simulink model "test_gps_01"  (Simulink 8.8)
settings: Solver=FixedStepDiscrete  StartTime=0.0  StopTime=10.0  FixedStep=0.001  RelTol=1e-3  EnableMultiTasking=on
InitFcn:
  | px4_ap1_mdl_callback('check_model');
libraries: px4_ap1_px4setup_lib x1, px4_ap1_gps_lib x1
settings Model: Creator=Privat  LastModifiedBy=Privat
settings OptimizationCC: ExpressionDepthLimit=2147483647  InitFltsAndDblsToZero=on  LifeSpan=1
settings DebuggingCC: SolverPrmCheckMsg=warning  InheritedTsInSrcMsg=none  StrictBusMsg=Warning
settings RTWCC: SystemTargetFile=px4_ap1.tlc  GenCodeOnly=on  GenerateMakefile=off
settings CodeAppCC: IgnoreCustomStorageClasses=off  CustomSymbolStrType=$N$R$M  InternalIdentifier=Classic
settings STFCustomTargetCC: ModelReferenceCompliant=off  IncludeMdlTerminateFcn=off  CombineOutputUpdateFcns=on  ERTCustomFileBanners=on  SupportContinuousTime=off  SupportNonInlinedSFcns=off  RemoveResetFunc=on  MATLABClassNameForMDSCustomization=Simulink.SoftwareTarget.ERTCustomization  CPPClassGenCompliant=on  GRTInterface=off  SystemTargetFile=px4_ap1.tlc
settings ERTTargetCC: MultiwordLength=2048  ModelReferenceCompliant=off  ParMdlRefBuildCompliant=off  CompOptLevelCompliant=off  ConcurrentExecutionCompliant=off  IncludeMdlTerminateFcn=off  ERTFirstTimeCompliant=off  ModelStepFunctionPrototypeControlCompliant=off  UseToolchainInfoCompliant=off  ERTSrcFileBannerTemplate=px4_ap1_code_template.cgt  ERTHdrFileBannerTemplate=px4_ap1_code_template.cgt  ERTDataSrcFileTemplate=px4_ap1_code_template.cgt  ERTDataHdrFileTemplate=px4_ap1_code_template.cgt  ERTCustomFileTemplate=px4_ap1_main.tlc  ConvertIfToSwitch=off  SuppressUnreachableDefaultCases=off

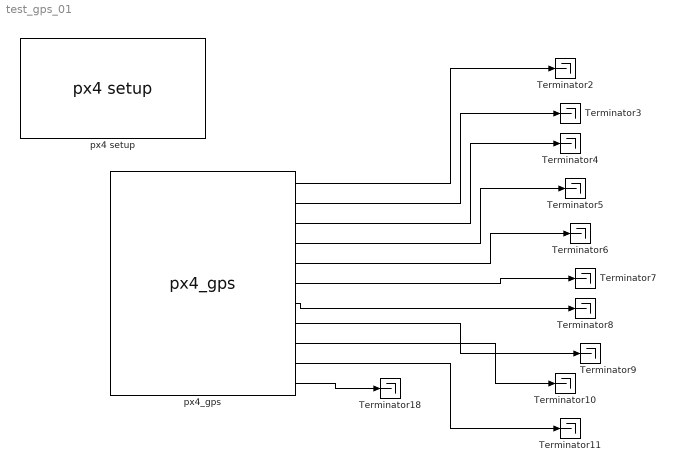
== system test_gps_01 ==
  Terminator{2..11,18} (11 alike) : Terminator
  px4 setup : px4_ap1_px4setup_lib/px4 setup  SampleTimeValue=0.001  cbBuild=on  cbUpload=off  cbPort=COM3  cpuLoad=off  debugmode=on
  px4_gps : px4_ap1_gps_lib/px4_gps  Description=Setup for PX4 native software  baud=9600  latlon=on  speed=on  course=on  time=on  date=on
  wires:
  px4_gps/1 -> Terminator2/1
  px4_gps/2 -> Terminator3/1
  px4_gps/3 -> Terminator4/1
  px4_gps/4 -> Terminator5/1
  px4_gps/5 -> Terminator6/1
  px4_gps/6 -> Terminator7/1
  px4_gps/7 -> Terminator8/1
  px4_gps/8 -> Terminator9/1
  px4_gps/9 -> Terminator10/1
  px4_gps/10 -> Terminator11/1
  px4_gps/11 -> Terminator18/1
